simulink model "adc4x16g_two_adcs"  (R2018a)
settings: Solver=VariableStepAuto  StartTime=0.0  StopTime=10.0  RelTol=1e-3
libraries: xbsIndex_r4 x12, xps_library x5
settings Model: Creator=wei  LastModifiedBy=wei

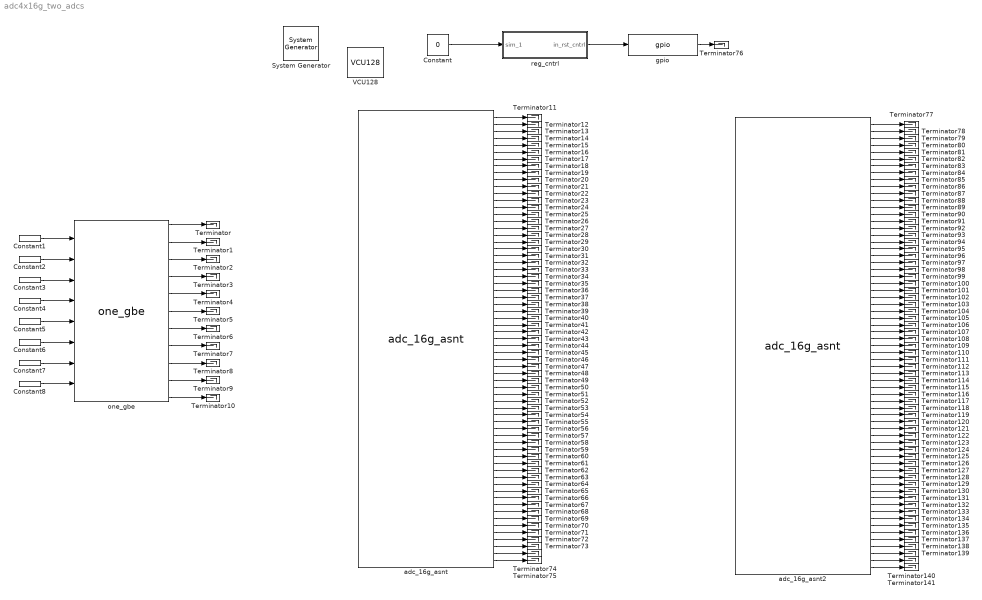
== system adc4x16g_two_adcs ==
  " System Generator" : xbsIndex_r4/ System Generator  Tag=genX  xilinxfamily=virtexuplusHBM  part=xcvu37p  speed=-2L-e  package=fsvh2892  synthesis_tool=XST  clock_wrapper=Clock Enables  directory=/home/wei/casper/VCU128_test/adc4x16_two_adcs/adc4x16g_two_adcs/sysgen  proj_type=Vivado  Synth_file=Vivado Synthesis Defaults  Impl_file=Vivado Implementation Defaults  testbench=off  simulink_period=1  sysclk_period=4  dcm_input_clock_period=10  incr_netlist=off  trim_vbits=Everywhere in SubSystem  dbl_ovrd=According to Block Masks  core_generation=According to Block Masks  run_coregen=off  deprecated_control=off  eval_field=0  block_type=sysgen
  Constant : Constant  Value=0
  Constant{1..2,4,7..8} (5 alike) : xbsIndex_r4/Constant  const=0  gui_display_data_type=Fixed-point  arith_type=Unsigned  n_bits=1  bin_pt=0  preci_type=Single  exp_width=8  frac_width=24  explicit_period=off  period=1  equ=P=C  opselect=C  inp2=PCIN>>17  opr=+  inp1=P  carry=CIN  dbl_ovrd=off  block_type=constant
  Constant3 : xbsIndex_r4/Constant  const=0  gui_display_data_type=Fixed-point  arith_type=Unsigned  n_bits=8  bin_pt=0  preci_type=Single  exp_width=8  frac_width=24  explicit_period=off  period=1  equ=P=C  opselect=C  inp2=PCIN>>17  opr=+  inp1=P  carry=CIN  dbl_ovrd=off  block_type=constant
  Constant5 : xbsIndex_r4/Constant  const=0  gui_display_data_type=Fixed-point  arith_type=Unsigned  n_bits=32  bin_pt=0  preci_type=Single  exp_width=8  frac_width=24  explicit_period=off  period=1  equ=P=C  opselect=C  inp2=PCIN>>17  opr=+  inp1=P  carry=CIN  dbl_ovrd=off  block_type=constant
  Constant6 : xbsIndex_r4/Constant  const=0  gui_display_data_type=Fixed-point  arith_type=Unsigned  n_bits=16  bin_pt=0  preci_type=Single  exp_width=8  frac_width=24  explicit_period=off  period=1  equ=P=C  opselect=C  inp2=PCIN>>17  opr=+  inp1=P  carry=CIN  dbl_ovrd=off  block_type=constant
  Terminator{,1..141} (142 alike) : Terminator
  VCU128 : xps_library/Platforms/VCU128  Tag=xps:xsg  hw_sys=VCU128:xcvu37p  clk_src=adc_clk  clk_rate=250  use_microblaze=on  sample_period=1  synthesis_tool=XST
      settings: SourceProductName=CASPER XPS Blockset
  adc_16g_asnt : xps_library/ADCs/adc_16g_asnt  Tag=xps:adc_4x16g_asnt  channel_sel=0
      settings: SourceProductName=CASPER XPS Blockset
  adc_16g_asnt2 : xps_library/ADCs/adc_16g_asnt  Tag=xps:adc_4x16g_asnt  channel_sel=3
      settings: SourceProductName=CASPER XPS Blockset
  gpio : xps_library/IO/gpio  Tag=xps:gpio  io_group_params_forwarded=off  io_group=ROACH:led  io_group_real=led  io_group_custom=0  io_dir=out  arith_type=Boolean  bitwidth=1  bin_pt=0  bit_index=0  sample_period=1  use_single_ended=off  use_ddr=off  reg_iob=on  reg_clk_phase=0  termination=None
      settings: SourceProductName=CASPER XPS Blockset
  one_gbe : xps_library/IO/one_gbe  Tag=xps:onegbe  local_en=on  dis_cpu_rx=off  dis_cpu_tx=off  cpu_promiscuous=on  local_mac=hex2dec('123456789abc')  local_ip=hex2dec('c0a8290a')  local_port=4321  local_gateway=1
      settings: SourceProductName=CASPER XPS Blockset
  reg_cntrl : Subsystem  Tag=xps:sw_reg  AncestorBlock=xps_library/Memory/software_register  mask(swreg){io_dir=From Processor, io_delay=0, init_val=0, sample_period=1, names=rst_cntrl, bitwidths=[1], bin_pts=0, arith_types=[2], sim_port=on, show_format=on}
      mask prompts: io_dir "I/O direction"; io_delay "I/O delay"; init_val "Initial Value"; sample_period "Sample period"; names "Bitfield names [msb...lsb]"; bitwidths "Bitfield widths"; bin_pts "Bitfield binary pts"; arith_types "Bitfield types, ufix=0, fix=1, bool=2"; sim_port "Provide sim input/output?"; show_format "Print format string?"
      mask help: A 32-bit software-accessible register. Can be divided into bitfields of varying widths and types using the fields in the block mask.
      mask init:
      | swreg_init(gcb)
      settings: AttributesFormatString=1input:b = 1 bits
      mask TypeOptions io_dir: To Processor | From Processor
      mask Callback io_dir:
      | mask_enables = get_param(gcb, 'MaskEnables');
      | mask_names = get_param(gcb, 'MaskNames');
      | if strcmp(get_param(gcb, 'io_dir'), 'To Processor'),
      |     mask_enables{ismember(mask_names, 'sample_period')} = 'off';
      | else
      |     mask_enables{ismember(mask_names, 'sample_period')} = 'on';
      | end
      | set_param(gcb, 'MaskEnables', mask_enables);
      mask DialogControl ParameterTabVar0 Prompt: Setup
  wires:
  reg_cntrl/1(in_rst_cntrl) -> gpio/1
  Constant/1 -> reg_cntrl/1(sim_1)
  one_gbe/1 -> Terminator/1
  one_gbe/2 -> Terminator1/1
  one_gbe/3 -> Terminator2/1
  one_gbe/4 -> Terminator3/1
  one_gbe/5 -> Terminator4/1
  one_gbe/6 -> Terminator5/1
  one_gbe/7 -> Terminator6/1
  one_gbe/8 -> Terminator7/1
  one_gbe/9 -> Terminator8/1
  one_gbe/10 -> Terminator9/1
  one_gbe/11 -> Terminator10/1
  Constant1/1 -> one_gbe/1
  Constant2/1 -> one_gbe/2
  Constant3/1 -> one_gbe/3
  Constant4/1 -> one_gbe/4
  Constant5/1 -> one_gbe/5
  Constant8/1 -> one_gbe/8
  Constant7/1 -> one_gbe/7
  Constant6/1 -> one_gbe/6
  adc_16g_asnt/65 -> Terminator75/1
  adc_16g_asnt/64 -> Terminator74/1
  adc_16g_asnt/63 -> Terminator73/1
  adc_16g_asnt/62 -> Terminator72/1
  adc_16g_asnt/61 -> Terminator71/1
  adc_16g_asnt/60 -> Terminator70/1
  adc_16g_asnt/59 -> Terminator69/1
  adc_16g_asnt/58 -> Terminator68/1
  adc_16g_asnt/57 -> Terminator67/1
  adc_16g_asnt/56 -> Terminator66/1
  adc_16g_asnt/55 -> Terminator65/1
  adc_16g_asnt/54 -> Terminator64/1
  adc_16g_asnt/53 -> Terminator63/1
  adc_16g_asnt/52 -> Terminator62/1
  adc_16g_asnt/51 -> Terminator61/1
  adc_16g_asnt/50 -> Terminator60/1
  adc_16g_asnt/49 -> Terminator59/1
  adc_16g_asnt/48 -> Terminator58/1
  adc_16g_asnt/47 -> Terminator57/1
  adc_16g_asnt/46 -> Terminator56/1
  adc_16g_asnt/45 -> Terminator55/1
  adc_16g_asnt/44 -> Terminator54/1
  adc_16g_asnt/43 -> Terminator53/1
  adc_16g_asnt/42 -> Terminator52/1
  adc_16g_asnt/41 -> Terminator51/1
  adc_16g_asnt/40 -> Terminator50/1
  adc_16g_asnt/39 -> Terminator49/1
  adc_16g_asnt/38 -> Terminator48/1
  adc_16g_asnt/37 -> Terminator47/1
  adc_16g_asnt/36 -> Terminator46/1
  adc_16g_asnt/35 -> Terminator45/1
  adc_16g_asnt/34 -> Terminator44/1
  adc_16g_asnt/33 -> Terminator43/1
  adc_16g_asnt/32 -> Terminator42/1
  adc_16g_asnt/31 -> Terminator41/1
  adc_16g_asnt/30 -> Terminator40/1
  adc_16g_asnt/29 -> Terminator39/1
  adc_16g_asnt/28 -> Terminator38/1
  adc_16g_asnt/27 -> Terminator37/1
  adc_16g_asnt/1 -> Terminator11/1
  adc_16g_asnt/2 -> Terminator12/1
  adc_16g_asnt/3 -> Terminator13/1
  adc_16g_asnt/4 -> Terminator14/1
  adc_16g_asnt/5 -> Terminator15/1
  adc_16g_asnt/6 -> Terminator16/1
  adc_16g_asnt/7 -> Terminator17/1
  adc_16g_asnt/8 -> Terminator18/1
  adc_16g_asnt/9 -> Terminator19/1
  adc_16g_asnt/10 -> Terminator20/1
  adc_16g_asnt/11 -> Terminator21/1
  adc_16g_asnt/12 -> Terminator22/1
  adc_16g_asnt/13 -> Terminator23/1
  adc_16g_asnt/14 -> Terminator24/1
  adc_16g_asnt/15 -> Terminator25/1
  adc_16g_asnt/16 -> Terminator26/1
  adc_16g_asnt/17 -> Terminator27/1
  adc_16g_asnt/18 -> Terminator28/1
  adc_16g_asnt/19 -> Terminator29/1
  adc_16g_asnt/20 -> Terminator30/1
  adc_16g_asnt/21 -> Terminator31/1
  adc_16g_asnt/22 -> Terminator32/1
  adc_16g_asnt/23 -> Terminator33/1
  adc_16g_asnt/24 -> Terminator34/1
  adc_16g_asnt/25 -> Terminator35/1
  adc_16g_asnt/26 -> Terminator36/1
  gpio/1 -> Terminator76/1
  adc_16g_asnt2/13 -> Terminator89/1
  adc_16g_asnt2/58 -> Terminator134/1
  adc_16g_asnt2/15 -> Terminator91/1
  adc_16g_asnt2/34 -> Terminator110/1
  adc_16g_asnt2/18 -> Terminator94/1
  adc_16g_asnt2/24 -> Terminator100/1
  adc_16g_asnt2/53 -> Terminator129/1
  adc_16g_asnt2/3 -> Terminator79/1
  adc_16g_asnt2/8 -> Terminator84/1
  adc_16g_asnt2/44 -> Terminator120/1
  adc_16g_asnt2/10 -> Terminator86/1
  adc_16g_asnt2/32 -> Terminator108/1
  adc_16g_asnt2/14 -> Terminator90/1
  adc_16g_asnt2/38 -> Terminator114/1
  adc_16g_asnt2/30 -> Terminator106/1
  adc_16g_asnt2/35 -> Terminator111/1
  adc_16g_asnt2/43 -> Terminator119/1
  adc_16g_asnt2/52 -> Terminator128/1
  adc_16g_asnt2/29 -> Terminator105/1
  adc_16g_asnt2/23 -> Terminator99/1
  adc_16g_asnt2/41 -> Terminator117/1
  adc_16g_asnt2/19 -> Terminator95/1
  adc_16g_asnt2/37 -> Terminator113/1
  adc_16g_asnt2/1 -> Terminator77/1
  adc_16g_asnt2/33 -> Terminator109/1
  adc_16g_asnt2/21 -> Terminator97/1
  adc_16g_asnt2/27 -> Terminator103/1
  adc_16g_asnt2/17 -> Terminator93/1
  adc_16g_asnt2/5 -> Terminator81/1
  adc_16g_asnt2/60 -> Terminator136/1
  adc_16g_asnt2/4 -> Terminator80/1
  adc_16g_asnt2/65 -> Terminator141/1
  adc_16g_asnt2/59 -> Terminator135/1
  adc_16g_asnt2/54 -> Terminator130/1
  adc_16g_asnt2/39 -> Terminator115/1
  adc_16g_asnt2/51 -> Terminator127/1
  adc_16g_asnt2/36 -> Terminator112/1
  adc_16g_asnt2/22 -> Terminator98/1
  adc_16g_asnt2/2 -> Terminator78/1
  adc_16g_asnt2/40 -> Terminator116/1
  adc_16g_asnt2/11 -> Terminator87/1
  adc_16g_asnt2/63 -> Terminator139/1
  adc_16g_asnt2/26 -> Terminator102/1
  adc_16g_asnt2/42 -> Terminator118/1
  adc_16g_asnt2/47 -> Terminator123/1
  adc_16g_asnt2/6 -> Terminator82/1
  adc_16g_asnt2/45 -> Terminator121/1
  adc_16g_asnt2/7 -> Terminator83/1
  adc_16g_asnt2/57 -> Terminator133/1
  adc_16g_asnt2/31 -> Terminator107/1
  adc_16g_asnt2/20 -> Terminator96/1
  adc_16g_asnt2/64 -> Terminator140/1
  adc_16g_asnt2/61 -> Terminator137/1
  adc_16g_asnt2/12 -> Terminator88/1
  adc_16g_asnt2/46 -> Terminator122/1
  adc_16g_asnt2/9 -> Terminator85/1
  adc_16g_asnt2/48 -> Terminator124/1
  adc_16g_asnt2/28 -> Terminator104/1
  adc_16g_asnt2/49 -> Terminator125/1
  adc_16g_asnt2/16 -> Terminator92/1
  adc_16g_asnt2/25 -> Terminator101/1
  adc_16g_asnt2/56 -> Terminator132/1
  adc_16g_asnt2/55 -> Terminator131/1
  adc_16g_asnt2/50 -> Terminator126/1
  adc_16g_asnt2/62 -> Terminator138/1

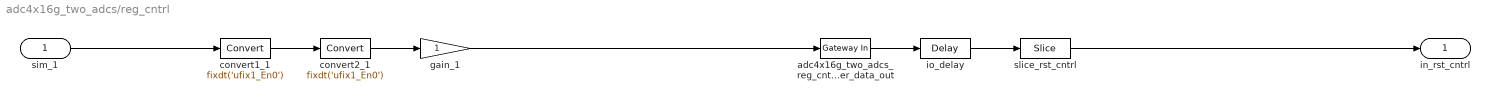
== system adc4x16g_two_adcs/reg_cntrl ==
  sim_1 : Inport
  adc4x16g_two_adcs_reg_cntrl_user_data_out : xbsIndex_r4/Gateway In  gui_display_data_type=Fixed-point  arith_type=Unsigned  n_bits=32  bin_pt=0  preci_type=Single  exp_width=8  frac_width=24  rows=1  columns=1  quantization="Round  (unbiased: +/- Inf)"  overflow=Saturate  period=1  UseAsADC=off  ADCChannel='1'  interface=None  automatic_assignment=on  address_offset=hex2dec('00')  intf_name=''  intf_description=''  default_value=0  timing_constraint=None  locs_specified=off  LOCs={}  io_standard={}  inherit_from_input=off  hdl_port=on  dbl_ovrd=off  block_type=gatewayin
  convert1_1 : DataTypeConversion  OutDataTypeStr=fixdt('ufix1_En0')  LockScale=on
  convert2_1 : DataTypeConversion  OutDataTypeStr=fixdt('ufix1_En0')  ConvertRealWorld=Stored Integer (SI)  LockScale=on
  gain_1 : Gain
  io_delay : xbsIndex_r4/Delay  rst=off  infoeditControl=Selection of Reset will increase slice count due to use of real FFs and instead of SRLs  en=off  latency=0  reg_retiming=on  dbl_ovrd=off  block_type=delay
  slice_rst_cntrl : xbsIndex_r4/Slice  nbits=1  boolean_output=on  mode=Lower Bit Location + Width  bit1=0  base1=MSB of Input  bit0=0  base0=LSB of Input  dbl_ovrd=off  block_type=slice
  in_rst_cntrl : Outport
  wires:
  adc4x16g_two_adcs_reg_cntrl_user_data_out/1 -> io_delay/1
  sim_1/1 -> convert1_1/1
  convert1_1/1 -> convert2_1/1
  convert2_1/1 -> gain_1/1
  gain_1/1 -> adc4x16g_two_adcs_reg_cntrl_user_data_out/1
  io_delay/1 -> slice_rst_cntrl/1
  slice_rst_cntrl/1 -> in_rst_cntrl/1
